simulink model "ex1alt"  (R2022a)
settings: Solver=VariableStepAuto  StartTime=0.0  StopTime=10.0  RelTol=1e-3
settings Model: Creator=Asus  LastModifiedBy=Asus

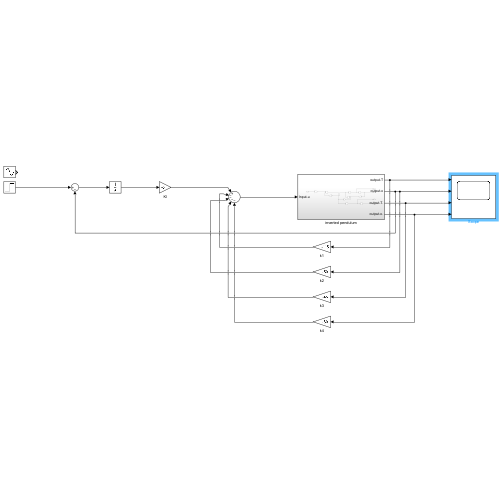
[thumbnail: Simulink's stored preview of the top-level diagram]
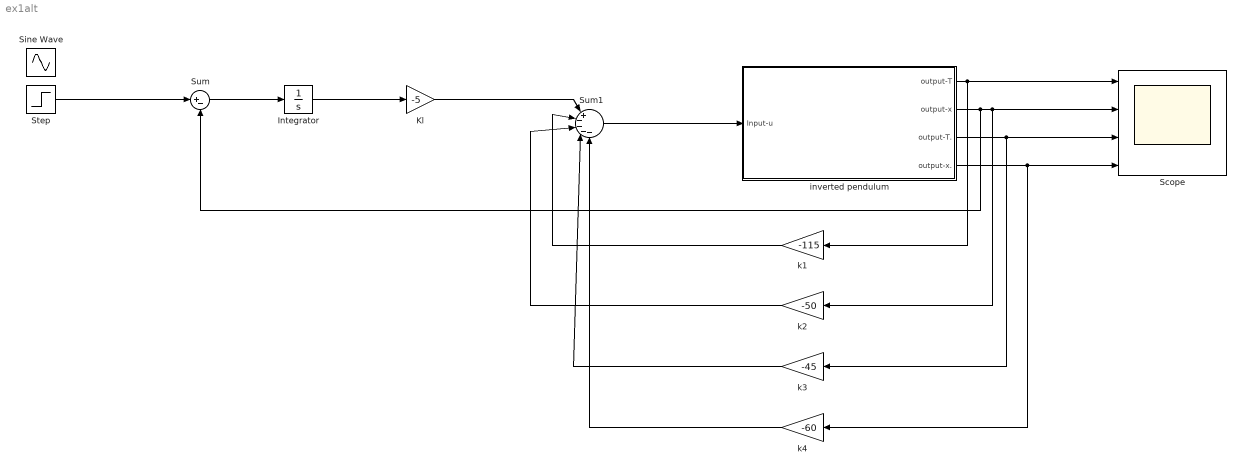
== system ex1alt ==
  Integrator : Integrator
  Kl : Gain  Gain=-5
  Scope : Scope  NumInputPorts=4
  Sine Wave : Sin  Frequency=2  SampleTime=0
  Step : Step  SampleTime=0
  Sum : Sum  Inputs=|+-
  Sum1 : Sum  Inputs=|+----
  inverted pendulum : Subsystem
  k1 : Gain  Gain=-115
  k2 : Gain  Gain=-50
  k3 : Gain  Gain=-45
  k4 : Gain  Gain=-60
  wires:
  Step/1 -> Sum/1
  Sum/1 -> Integrator/1
  Integrator/1 -> Kl/1
  Kl/1 -> Sum1/1
  Sum1/1 -> inverted pendulum/1(Input-u)
  k1/1 -> Sum1/2
  k2/1 -> Sum1/3
  k3/1 -> Sum1/4
  k4/1 -> Sum1/5
  inverted pendulum/2(output-x) -> Sum/2, k2/1, Scope/2
  inverted pendulum/1(output-T) -> k1/1, Scope/1
  inverted pendulum/3(output-T.) -> k3/1, Scope/3
  inverted pendulum/4(output-x.) -> k4/1, Scope/4

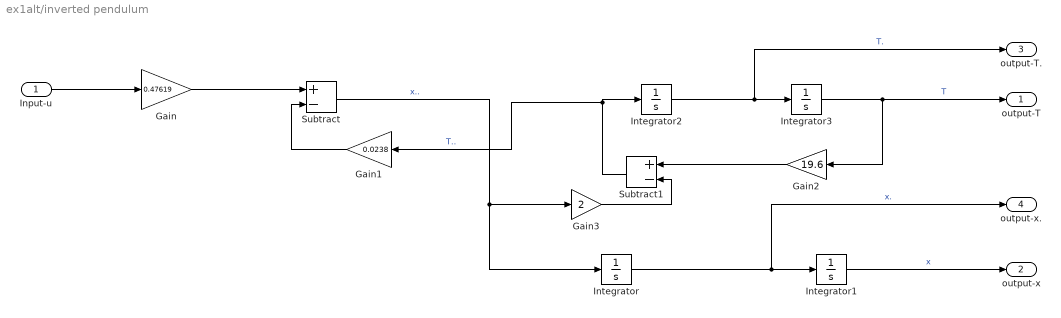
== system ex1alt/inverted pendulum ==
  Input-u : Inport
  Gain : Gain  Gain=0.47619
  Gain1 : Gain  Gain=0.0238
  Gain2 : Gain  Gain=19.6
  Gain3 : Gain  Gain=2
  Integrator{,1..3} (4 alike) : Integrator
  Subtract : Sum  Inputs=+-
  Subtract1 : Sum  Inputs=+-
  output-T : Outport
  output-x : Outport  Port=2
  output-T. : Outport  Port=3
  output-x. : Outport  Port=4
  wires:
  Input-u/1 -> Gain/1
  Gain/1 -> Subtract/1
  Integrator/1 -> output-x./1, Integrator1/1  "x."
  Subtract/1 -> Gain3/1, Integrator/1  "x.."
  Integrator2/1 -> output-T./1, Integrator3/1  "T."
  Integrator1/1 -> output-x/1  "x"
  Integrator3/1 -> Gain2/1, output-T/1  "T"
  Gain1/1 -> Subtract/2
  Gain2/1 -> Subtract1/1
  Subtract1/1 -> Gain1/1, Integrator2/1  "T.."
  Gain3/1 -> Subtract1/2
